simulink model "ASD"  (R2018a)
settings: configuration reference "cs_ert" (kept outside this file)
settings Model: DataDictionary=ASD.sldd  Creator=zhoutinglin  LastModifiedBy=zhoutinglin

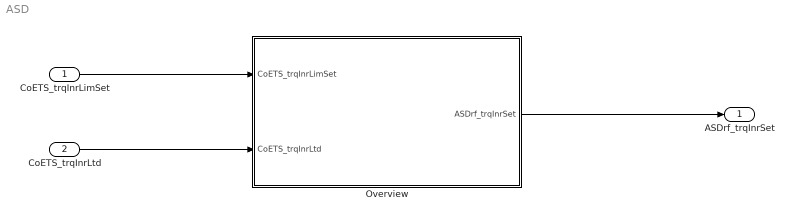
== system ASD ==
  CoETS_trqInrLimSet : Inport
  CoETS_trqInrLtd : Inport  Port=2
  Overview : Subsystem
  ASDrf_trqInrSet : Outport
  wires:
  CoETS_trqInrLimSet/1 -> Overview/1(CoETS_trqInrLimSet)
  CoETS_trqInrLtd/1 -> Overview/2(CoETS_trqInrLtd)
  Overview/1(ASDrf_trqInrSet) -> ASDrf_trqInrSet/1

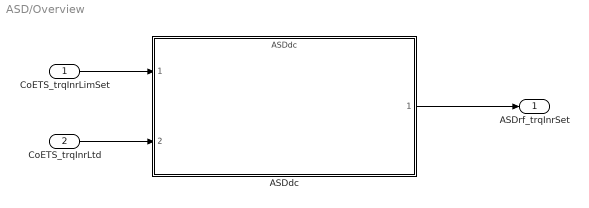
== system ASD/Overview ==
  CoETS_trqInrLimSet : Inport
  CoETS_trqInrLtd : Inport  Port=2
  ASDdc : ModelReference  ModelNameDialog=ASDdc  SimulationMode=Normal  ModelReferenceVersion=1.2
  ASDrf_trqInrSet : Outport
  wires:
  CoETS_trqInrLimSet/1 -> ASDdc/1
  CoETS_trqInrLtd/1 -> ASDdc/2
  ASDdc/1 -> ASDrf_trqInrSet/1
